simulink model "detumbling"  (R2021b)
settings: Solver=VariableStepAuto  StartTime=0.0  StopTime=T_det  RelTol=1e-6
values from neighbouring files (symbols this model uses):
  A0 = A_end    [Project.m]
  C = 1*eye(3)    [Project.m]
  om_0 = [0.22 0.26 0.22]    [Project.m]
  pointing_accuracy = 0.5    [Project.m]
  Q = eye(3)*1e-8    [Project.m]
  R = eye(3) + sin(ang)*axis_skewed + (1-cos(ang))*axis_skewed*axis_skewed    [Project.m]
  S_0 = eye(3)    [Project.m]
  sigma_b = 0.3*pi/180/3600/sqrt(Ts)    [Project.m]
  sigma_n = 0.15*pi/180/60/sqrt(Ts)    [Project.m]
  T_F = 50e-3    (= 0.05)    [Project.m]
  T_max = diag([T_max_1;T_max_2;T_max_3])    [Project.m]
  T_max_1 = 2*c*F*sind(15)    [Project.m]
  T_max_2 = 2*c*F*cosd(15)    [Project.m]
  T_max_3 = 2*(x*F*cosd(15)-x*F*sind(15))    [Project.m]
  T_R = 10e-3    (= 0.01)    [Project.m]
  Ts = 1/f    (= 0.00381679389313)    [Project.m]
undefined symbols (not defined in the file or in its folder): J
settings Model: Creator=miche  LastModifiedBy=hp
settings SolverCC: AlgebraicLoopSolver=TrustRegion
settings DataIOCC: ReturnWorkspaceOutputs=off
settings DebuggingCC: SFMachineParentedDataDiag=warning  ArithmeticOperatorsInVariantConditions=warning
settings SFSimCC: CustomCodeUndefinedFunction=UseInterfaceOnly

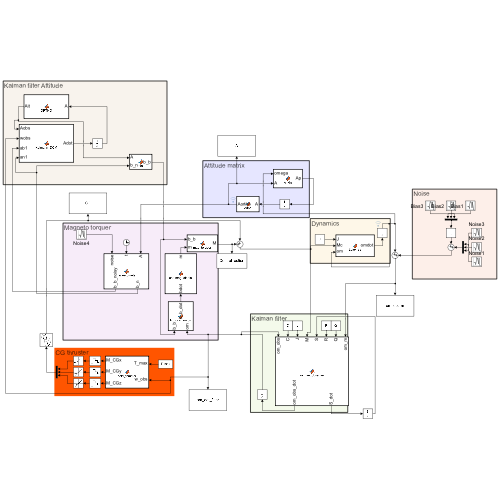
[thumbnail: Simulink's stored preview of the top-level diagram]
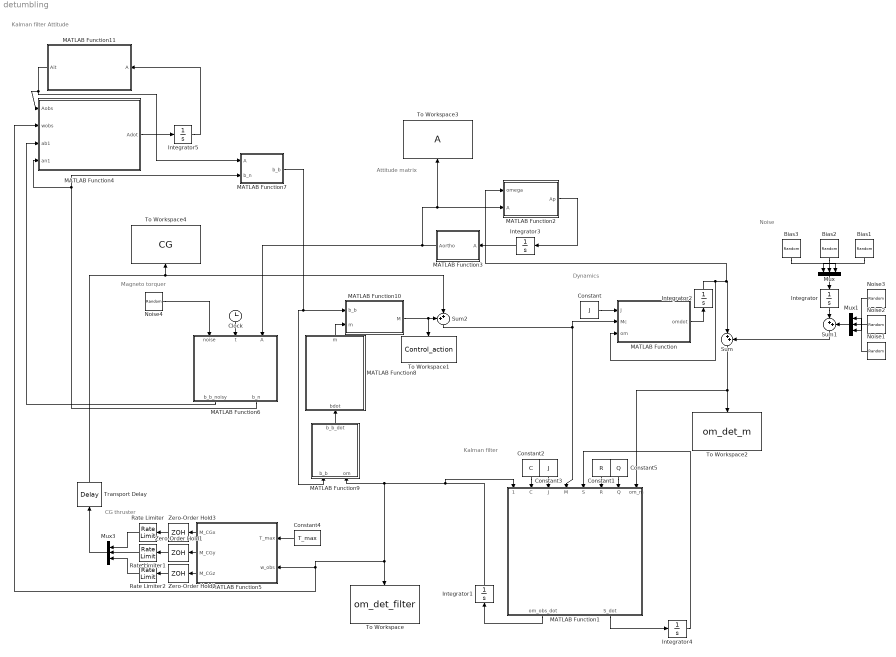
== system detumbling ==
  note: Kalman filter Attitude
  note: CG thruster
  note: Magneto torquer
  note: Dynamics
  note: Kalman filter
  note: Noise
  note: Attitude matrix
  Bias1 : RandomNumber  Variance=sigma_b^2  Seed=1  SampleTime=Ts
  Bias2 : RandomNumber  Variance=sigma_b^2  Seed=2  SampleTime=Ts
  Bias3 : RandomNumber  Variance=sigma_b^2  Seed=3  SampleTime=Ts
  Clock : Clock
  Constant : Constant  Value=J
  Constant1 : Constant  Value=R
  Constant2 : Constant  Value=C
  Constant3 : Constant  Value=J
  Constant4 : Constant  Value=T_max
  Constant5 : Constant  Value=Q
  Integrator : Integrator
  Integrator1 : Integrator  InitialCondition=om_0
  Integrator2 : Integrator  InitialCondition=om_0
  Integrator3 : Integrator  InitialCondition=A0
  Integrator4 : Integrator  InitialCondition=S_0
  Integrator5 : Integrator  InitialCondition=A0
  MATLAB Function : MATLAB Function  TreatAsAtomicUnit=on
  MATLAB Function1 : MATLAB Function  TreatAsAtomicUnit=on
  MATLAB Function10 : MATLAB Function  TreatAsAtomicUnit=on
  MATLAB Function11 : MATLAB Function  TreatAsAtomicUnit=on
  MATLAB Function2 : MATLAB Function  TreatAsAtomicUnit=on
  MATLAB Function3 : MATLAB Function  TreatAsAtomicUnit=on
  MATLAB Function4 : MATLAB Function  TreatAsAtomicUnit=on
  MATLAB Function5 : MATLAB Function  TreatAsAtomicUnit=on
  MATLAB Function6 : MATLAB Function  TreatAsAtomicUnit=on
  MATLAB Function7 : MATLAB Function  TreatAsAtomicUnit=on
  MATLAB Function8 : MATLAB Function  TreatAsAtomicUnit=on
  MATLAB Function9 : MATLAB Function  TreatAsAtomicUnit=on
  Mux : Mux  Inputs=3
  Mux1 : Mux  Inputs=3
  Mux3 : Mux  Inputs=3
  Noise1 : RandomNumber  Variance=sigma_n^2  Seed=4  SampleTime=Ts
  Noise2 : RandomNumber  Variance=sigma_n^2  Seed=5  SampleTime=Ts
  Noise3 : RandomNumber  Variance=sigma_n^2  Seed=6  SampleTime=Ts
  Noise4 : RandomNumber  Variance=(pointing_accuracy*pi/180)^2  Seed=4  SampleTime=Ts
  Rate Limiter : RateLimiter  RisingSlewLimit=T_max_1/T_R  FallingSlewLimit=-T_max_1/T_F
  Rate Limiter1 : RateLimiter  RisingSlewLimit=T_max_2/T_R  FallingSlewLimit=-T_max_2/T_F
  Rate Limiter2 : RateLimiter  RisingSlewLimit=T_max_3/T_R  FallingSlewLimit=-T_max_3/T_F
  Sum : Sum  Inputs=|++
  Sum1 : Sum  Inputs=|++
  Sum2 : Sum  Inputs=++|
  To Workspace : ToWorkspace  VariableName=om_det_filter  SaveFormat=Timeseries  SampleTime=-1
  To Workspace1 : ToWorkspace  VariableName=Control_action  SaveFormat=Timeseries  SampleTime=-1
  To Workspace2 : ToWorkspace  VariableName=om_det_m  SaveFormat=Timeseries  SampleTime=-1
  To Workspace3 : ToWorkspace  VariableName=A  SaveFormat=Timeseries  SampleTime=-1
  To Workspace4 : ToWorkspace  VariableName=CG  SaveFormat=Timeseries  SampleTime=-1
  Transport Delay : TransportDelay  DelayTime=5e-3
  Zero-Order Hold1 : ZeroOrderHold  SampleTime=0.05
  Zero-Order Hold2 : ZeroOrderHold  SampleTime=0.05
  Zero-Order Hold3 : ZeroOrderHold  SampleTime=0.05
  wires:
  MATLAB Function9/1(b_b_dot) -> MATLAB Function8/1(bdot)
  Clock/1 -> MATLAB Function6/2(t)
  Noise1/1 -> Mux1/1
  Noise3/1 -> Mux1/3
  Noise2/1 -> Mux1/2
  MATLAB Function1/1(om_obs_dot) -> Integrator1/1
  MATLAB Function3/1(Aortho) -> MATLAB Function6/3(A), To Workspace3/1, MATLAB Function2/2(A)
  Integrator2/1 -> MATLAB Function/3(om), MATLAB Function2/1(omega), Sum/1
  Integrator3/1 -> MATLAB Function3/1(A)
  MATLAB Function2/1(Ap) -> Integrator3/1
  Bias2/1 -> Mux/2
  Mux/1 -> Integrator/1
  Bias3/1 -> Mux/3
  Bias1/1 -> Mux/1
  Integrator/1 -> Sum1/1
  Mux1/1 -> Sum1/2
  Sum1/1 -> Sum/2
  Constant/1 -> MATLAB Function/1(J)
  Sum/1 -> MATLAB Function1/8(om_m), To Workspace2/1
  Constant2/1 -> MATLAB Function1/2(C)
  Constant3/1 -> MATLAB Function1/3(J)
  MATLAB Function4/1(Adot) -> Integrator5/1
  MATLAB Function8/1(m) -> MATLAB Function10/2(m)
  MATLAB Function10/1(M) -> To Workspace1/1, Sum2/1
  Sum2/1 -> MATLAB Function1/4(M), MATLAB Function/2(Mc)
  Noise4/1 -> MATLAB Function6/1(noise)
  MATLAB Function6/1(b_b_noisy) -> MATLAB Function4/3(ab1)
  Integrator5/1 -> MATLAB Function11/1(A)
  MATLAB Function11/1(Ait) -> MATLAB Function7/1(A), MATLAB Function4/1(Aobs)
  MATLAB Function7/1(b_b) -> MATLAB Function10/1(b_b), MATLAB Function9/1(b_b)
  MATLAB Function/1(omdot) -> Integrator2/1
  Constant4/1 -> MATLAB Function5/1(T_max)
  MATLAB Function6/2(b_n) -> MATLAB Function7/2(b_n), MATLAB Function4/4(an1)
  Rate Limiter/1 -> Mux3/1
  Rate Limiter1/1 -> Mux3/2
  Rate Limiter2/1 -> Mux3/3
  Mux3/1 -> Transport Delay/1
  Transport Delay/1 -> To Workspace4/1, Sum2/2
  Zero-Order Hold3/1 -> Rate Limiter/1
  MATLAB Function5/1(M_CGx) -> Zero-Order Hold3/1
  Zero-Order Hold1/1 -> Rate Limiter1/1
  MATLAB Function5/2(M_CGy) -> Zero-Order Hold1/1
  Zero-Order Hold2/1 -> Rate Limiter2/1
  MATLAB Function5/3(M_CGz) -> Zero-Order Hold2/1
  Integrator1/1 -> MATLAB Function9/2(om), MATLAB Function5/2(w_obs), MATLAB Function4/2(wobs), To Workspace/1, MATLAB Function1/1(om_obs)
  MATLAB Function1/2(S_dot) -> Integrator4/1
  Integrator4/1 -> MATLAB Function1/5(S)
  Constant5/1 -> MATLAB Function1/7(Q)
  Constant1/1 -> MATLAB Function1/6(R)

== matlab function detumbling/MATLAB Function10 ==
  data: b_b input; m input; M output
function M=mag_torquer(b_b,m)
M=cross(m,b_b);
end

== matlab function detumbling/MATLAB Function4 ==
  data: Aobs input; wobs input; ab1 input; an1 input; Adot output
function Adot = Kalmann_DCM(Aobs,wobs,ab1,an1)

ab1=ab1/norm(ab1);
an1=an1/norm(an1);

k1=0.1;

wmatr=[0, -wobs(3), wobs(2); wobs(3),0,-wobs(1);-wobs(2),wobs(1),0];
alfa=k1*(cross(ab1,Aobs*an1));
alfam=[0, -alfa(3), alfa(2); alfa(3),0,-alfa(1);-alfa(2),alfa(1),0];
Adot=-(wmatr+alfam)*Aobs;

== matlab function detumbling/MATLAB Function11 ==
  data: A input; Ait output
function Ait   = ORTHO(A)

Ait= A;
for k=1:15
    
    Ait= Ait*3/2-Ait*(Ait')*Ait/2;
    
end

% vec=A(:,1);
end

== matlab function detumbling/MATLAB Function1 ==
  data: om_obs input; C input; J input; M input; S input; R input; Q input; om_m input; om_obs_dot output; S_dot output
function [om_obs_dot,S_dot] = kalman_observer(om_obs,C,J,M,S,R,Q,om_m)

L = S*C'*inv(R);
K_x=(J(2)-J(3))/J(1);
K_y=(J(3)-J(1))/J(2);
K_z=(J(1)-J(2))/J(3);
A = [0 K_x*om_obs(3) K_x*om_obs(2); K_y*om_obs(3) 0 K_y*om_obs(1); K_z*om_obs(2) K_z*om_obs(1) 0];
% Reconstruction of the state:
L_Dy=L*[(om_m(1)-C(1,1)*om_obs(1));
    (om_m(2)-C(2,2)*om_obs(2));
    (om_m(3)-C(3,3)*om_obs(3))];

om_obs_dot_x=K_x*om_obs(2)*om_obs(3)+M(1)/J(1)+L_Dy(1);
om_obs_dot_y=K_y*om_obs(1)*om_obs(3)+M(2)/J(2)+L_Dy(2);
om_obs_dot_z=K_z*om_obs(2)*om_obs(1)+M(3)/J(3)+L_Dy(3);
om_obs_dot=[om_obs_dot_x om_obs_dot_y om_obs_dot_z];
S_dot = S*A' + A*S +Q- S*C'*inv(R)*C*S;

end

== matlab function detumbling/MATLAB Function ==
  data: J input; Mc input; om input; omdot output
function omdot  = Euler_eq(J,Mc,om)

% Euler equations:

omdot_x=(J(2)-J(3))/J(1)*om(2)*om(3)+Mc(1)/J(1);
omdot_y=(J(3)-J(1))/J(2)*om(1)*om(3)+Mc(2)/J(2);
omdot_z=(J(1)-J(2))/J(3)*om(2)*om(1)+Mc(3)/J(3);
omdot=[omdot_x omdot_y omdot_z];
end

== matlab function detumbling/MATLAB Function2 ==
  data: omega input; Ap output; A input
function Ap = A_kin(omega,A)

Ap=-[0, -omega(3), omega(2);omega(3), 0, -omega(1);-omega(2), omega(1), 0]*A;

end

== matlab function detumbling/MATLAB Function3 ==
  data: A input; Aortho output
function Aortho  = ortho(A)

% Orthonomalization process
for i=1:10
    A=3/2*A-A*(A')*A*1/2;
end
Aortho=A;
end

== matlab function detumbling/MATLAB Function5 ==
  data: T_max input; w_obs input; M_CGx output; M_CGy output; M_CGz output
function [M_CGx,M_CGy,M_CGz]  = cold_thruster(T_max,w_obs)
% Bang-bang configuration:
% M_CG=-T_max*sign(w_obs);
Matr=zeros(3);
w_mod=abs(w_obs);
[~,i]=max(w_mod);
Matr(i,i)=T_max(i,i);
if w_mod(i)>5e-4
M_CG=-Matr*sign(w_obs);
else
 M_CG=zeros(3,1);
 
end
  M_CGx=M_CG(1);
  M_CGy=M_CG(2);
  M_CGz=M_CG(3);

== matlab function detumbling/MATLAB Function7 ==
  data: A input; b_b output; b_n input
function b_b = fcn(A,b_n)
b_b=A*b_n;

== matlab function detumbling/MATLAB Function6 ==
  data: noise input; t input; A input; b_b_noisy output; b_n output
function [b_b_noisy,b_n]   = magnetometer(noise,t,A)

%Magnetic dipole vector of the Earth:

m_hat= [sind(11.5)*cos(7.2722e-05*t);
        sind(11.5)*sin(7.2722e-05*t);
        cosd(11.5)];
    
%Parameters:

g10=-29615e-9;
g11=-1728e-9;
h11=5186e-9;
H0=sqrt(g10^2+g11^2+h11^2);
R=6378;

% Position vector of the satellite:

r=42164*[cos(7.2722e-05*t);sin(7.2722e-05*t);sin(7.2722e-05*t)];

% Vector of the magnetic field of the Earth:

b_n= R^3*H0/(norm(r)^3)*(3*dot(m_hat,r'/norm(r))*r/norm(r)-m_hat); 

% Error matrix:

err=noise;
Aerr= [cos(err)*cos(err), cos(err)*sin(err)*sin(err)+sin(err)*cos(err), -cos(err)*sin(err)*cos(err)+sin(err)*sin(err);
            -sin(err)*cos(err), -sin(err)*sin(err)*sin(err)+cos(err)*cos(err), sin(err)*sin(err)*cos(err)+cos(err)*sin(err);
            sin(err), -cos(err)*sin(err), cos(err)*cos(err)];
        
% Vector of the magnetic field of the Earth in th local frame:
A1=Aerr*A;
b_b_noisy=A1*b_n;




end

== matlab function detumbling/MATLAB Function8 ==
  data: bdot input; m output
function m =sat_mag_dipole(bdot)
% I have only 1 magnetic torquer.
m=-1.2*sign(bdot);
m(3)=0;
m(2)=0;


end

== matlab function detumbling/MATLAB Function9 ==
  data: b_b input; b_b_dot output; om input
function b_b_dot=b_b_dynamics(b_b,om)
b_b_dot=cross(b_b,om);
 end
